simulink model "TiltRotorQuad"  (R2022b)
settings: Solver=VariableStepAuto  StartTime=0.0  StopTime=10  RelTol=1e-3
values from neighbouring files (symbols this model uses):
  k = 7.075135827e-05    [QuadSimParameters.mat]
undefined symbols (not defined in the file or in its folder): X, Y, Z
libraries: sm_lib x46, nesl_utility x25
(part 1 of 3)
settings Model: Creator=sudip  LastModifiedBy=sudip

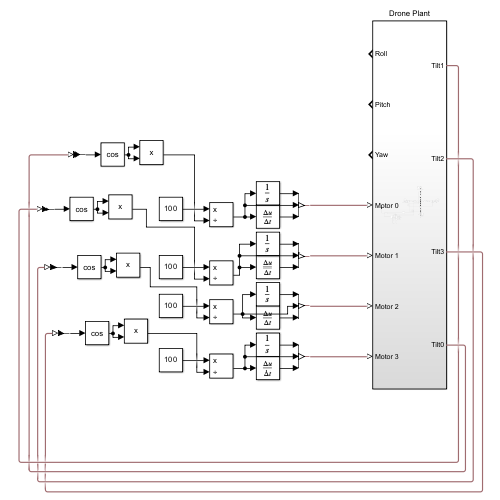
[thumbnail: Simulink's stored preview of the top-level diagram]
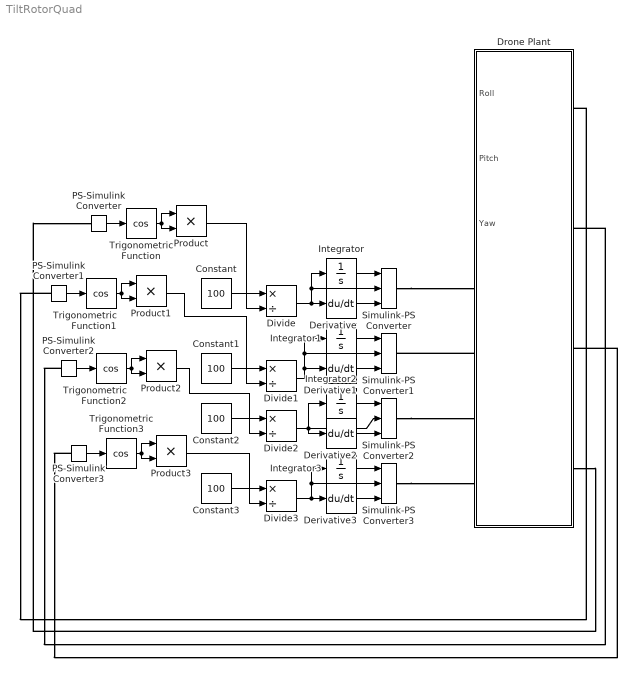
== system TiltRotorQuad ==
  Constant{,1..3} (4 alike) : Constant  Value=100
  Derivative{,1..3} (4 alike) : Derivative
  Divide{,1..3} (4 alike) : Product  Inputs=*/
  Drone Plant : Subsystem
  Integrator{,1..3} (4 alike) : Integrator
  PS-Simulink Converter{,1..3} (4 alike) : nesl_utility/PS-Simulink Converter  PhysicalDomain=network_engine_domain  SubClassName=ps_output  LeftPortType=input  RightPortType=output  PseudoPeriodic=off  Frequencies=[]  VectorFormat=inherit  Unit=inherit  AffineConversion=off
  Product{,1..3} (4 alike) : Product
  Simulink-PS Converter{,1..3} (4 alike) : nesl_utility/Simulink-PS Converter  PhysicalDomain=network_engine_domain  SubClassName=ps_input  LeftPortType=input  RightPortType=output  PseudoPeriodic=off  Frequencies=[]  NoiseDistribution=none  NoiseParameters=[]  Unit=1  AffineConversion=off  FilteringAndDerivatives=provide  SimscapeFilterOrder=1  InputFilterTimeConstant=0.001  UdotUserProvided=2
  Trigonometric Function{,1..3} (4 alike) : Trigonometry  Operator=cos
  wires:
  Derivative/1 -> Simulink-PS Converter/3
  Integrator/1 -> Simulink-PS Converter/1
  Integrator1/1 -> Simulink-PS Converter1/1
  Derivative1/1 -> Simulink-PS Converter1/3
  Derivative2/1 -> Simulink-PS Converter2/3
  Integrator2/1 -> Simulink-PS Converter2/1
  Integrator3/1 -> Simulink-PS Converter3/1
  Derivative3/1 -> Simulink-PS Converter3/3
  PS-Simulink Converter/1 -> Trigonometric Function/1
  Trigonometric Function/1 -> Product/1, Product/2
  Product/1 -> Divide/2
  Constant/1 -> Divide/1
  Divide/1 -> Derivative/1, Integrator/1, Simulink-PS Converter/2
  Product1/1 -> Divide1/2
  Trigonometric Function1/1 -> Product1/2, Product1/1
  PS-Simulink Converter1/1 -> Trigonometric Function1/1
  Constant1/1 -> Divide1/1
  Divide1/1 -> Derivative1/1, Integrator1/1, Simulink-PS Converter1/2
  Product2/1 -> Divide2/2
  Trigonometric Function2/1 -> Product2/2, Product2/1
  PS-Simulink Converter2/1 -> Trigonometric Function2/1
  Constant2/1 -> Divide2/1
  Divide2/1 -> Integrator2/1, Derivative2/1, Simulink-PS Converter2/2
  PS-Simulink Converter3/1 -> Trigonometric Function3/1
  Trigonometric Function3/1 -> Product3/1, Product3/2
  Constant3/1 -> Divide3/1
  Divide3/1 -> Integrator3/1, Simulink-PS Converter3/2, Derivative3/1
  Product3/1 -> Divide3/2
  connections:
  Simulink-PS Converter/RConn1 -- Drone Plant/RConn1
  Drone Plant/RConn2 -- Simulink-PS Converter1/RConn1
  Simulink-PS Converter2/RConn1 -- Drone Plant/RConn3
  Simulink-PS Converter3/RConn1 -- Drone Plant/RConn4
  Drone Plant/LConn4 -- PS-Simulink Converter/LConn1
  PS-Simulink Converter1/LConn1 -- Drone Plant/LConn1
  PS-Simulink Converter2/LConn1 -- Drone Plant/LConn2
  PS-Simulink Converter3/LConn1 -- Drone Plant/LConn3
